simulink model "QN1F_induction_motor_v10"  (R2025b)
settings: Solver=ode45  StartTime=0.0  StopTime=10  RelTol=1e-3
PreLoadFcn:
  | run('QN1F_params_v10.m')
StopFcn:
  | QN1F_plot_results_v10
values from neighbouring files (symbols this model uses):
  B = 2.0e-5    (= 2e-05)    [QN1F_params_v10.m]
  f_max = n_max*pole_pairs/60    (= 400)    [QN1F_params_v10.m]
  I_rated = 10    [QN1F_params_v10.m]
  J = 2.5e-3    (= 0.0025)    [QN1F_params_v10.m]
  K_slip = T_rated/s_ref_model    (= 115)    [QN1F_params_v10.m]
  Kp_f = 0.05    [QN1F_params_v10.m]
  n_max = 24000    [QN1F_params_v10.m]
  n_ref = n_rated    (= 18000)    [QN1F_params_v10.m]
  pole_pairs = 1    [QN1F_params_v10.m]
  T_cut_amp = 0.15    [QN1F_params_v10.m]
  T_cut_mean = 1.0    (= 1)    [QN1F_params_v10.m]
  t_cut_start = 4.0    (= 4)    [QN1F_params_v10.m]
  T_rated = 2.3    [QN1F_params_v10.m]
  tau_T = 0.05    [QN1F_params_v10.m]
  w_tooth = 2*pi*f_tooth    (= 3769.91118431)    [QN1F_params_v10.m]
settings Model: Creator=jaxja  LastModifiedBy=jaxja
settings DataIOCC: ReturnWorkspaceOutputs=off

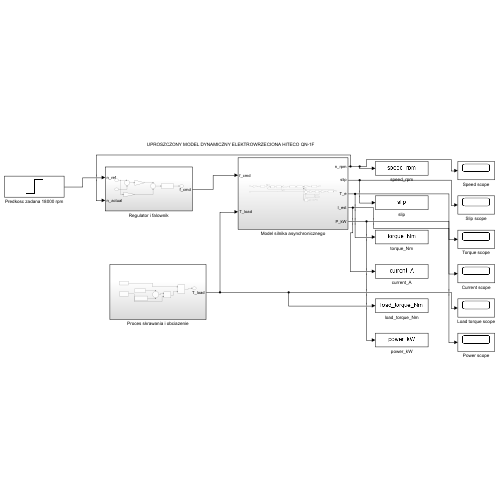
[thumbnail: Simulink's stored preview of the top-level diagram]
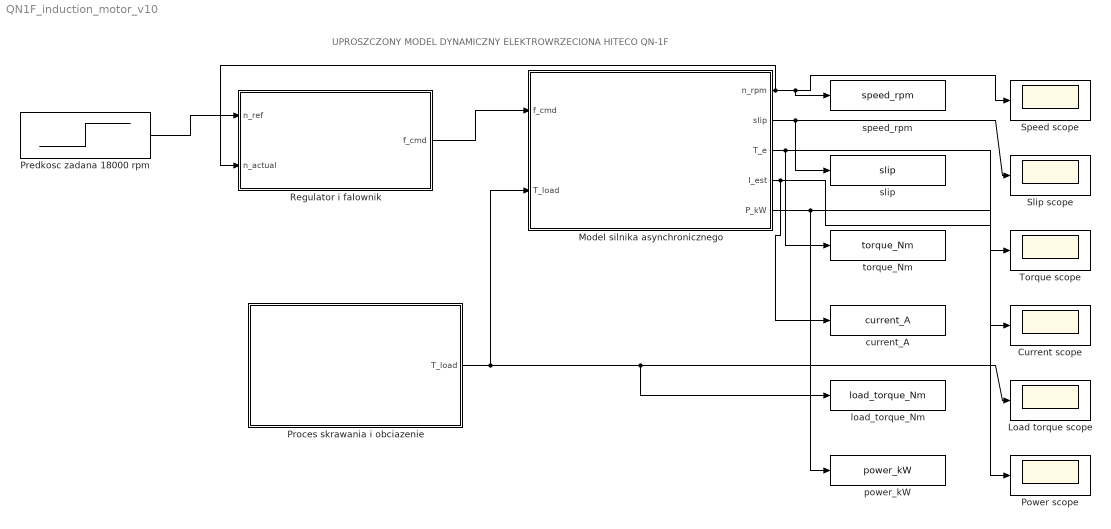
== system QN1F_induction_motor_v10 ==
  note: UPROSZCZONY MODEL DYNAMICZNY ELEKTROWRZECIONA HITECO QN-1F
  Current scope : Scope
  Load torque scope : Scope
  Model silnika asynchronicznego : Subsystem
  Power scope : Scope
  Predkosc zadana 18000 rpm : Step  Time=0.2  After=n_ref  SampleTime=0
  Proces skrawania i obciazenie : Subsystem
  Regulator i falownik : Subsystem
  Slip scope : Scope
  Speed scope : Scope
  Torque scope : Scope
  current_A : ToWorkspace  VariableName=current_A  SaveFormat=Timeseries  SampleTime=-1
  load_torque_Nm : ToWorkspace  VariableName=load_torque_Nm  SaveFormat=Timeseries  SampleTime=-1
  power_kW : ToWorkspace  VariableName=power_kW  SaveFormat=Timeseries  SampleTime=-1
  slip : ToWorkspace  VariableName=slip  SaveFormat=Timeseries  SampleTime=-1
  speed_rpm : ToWorkspace  VariableName=speed_rpm  SaveFormat=Timeseries  SampleTime=-1
  torque_Nm : ToWorkspace  VariableName=torque_Nm  SaveFormat=Timeseries  SampleTime=-1
  wires:
  Predkosc zadana 18000 rpm/1 -> Regulator i falownik/1(n_ref)
  Regulator i falownik/1(f_cmd) -> Model silnika asynchronicznego/1(f_cmd)
  Proces skrawania i obciazenie/1(T_load) -> load_torque_Nm/1, Load torque scope/1, Model silnika asynchronicznego/2(T_load)
  Model silnika asynchronicznego/1(n_rpm) -> speed_rpm/1, Speed scope/1, Regulator i falownik/2(n_actual)
  Model silnika asynchronicznego/2(slip) -> slip/1, Slip scope/1
  Model silnika asynchronicznego/3(T_e) -> torque_Nm/1, Torque scope/1
  Model silnika asynchronicznego/4(I_est) -> current_A/1, Current scope/1
  Model silnika asynchronicznego/5(P_kW) -> power_kW/1, Power scope/1

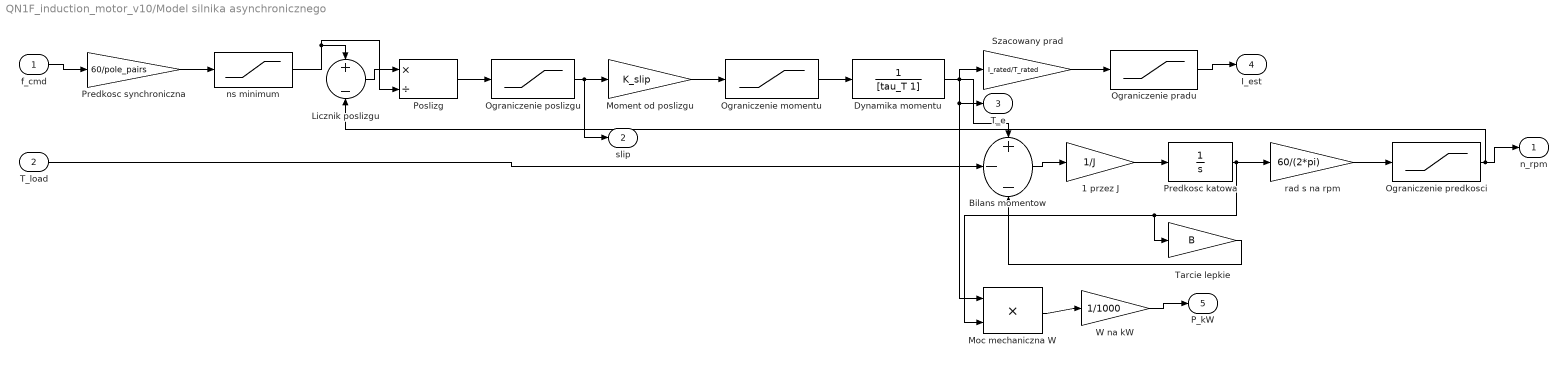
== system QN1F_induction_motor_v10/Model silnika asynchronicznego ==
  f_cmd : Inport
  T_load : Inport  Port=2
  1 przez J : Gain  Gain=1/J
  Bilans momentow : Sum  Inputs=+--
  Dynamika momentu : TransferFcn  Numerator=1  Denominator=[tau_T 1]
  Licznik poslizgu : Sum  Inputs=+-
  Moc mechaniczna W : Product
  Moment od poslizgu : Gain  Gain=K_slip
  Ograniczenie momentu : Saturate  UpperLimit=T_rated  LowerLimit=0
  Ograniczenie poslizgu : Saturate  UpperLimit=1  LowerLimit=0
  Ograniczenie pradu : Saturate  UpperLimit=I_rated  LowerLimit=0
  Ograniczenie predkosci : Saturate  UpperLimit=n_max  LowerLimit=0
  Poslizg : Product  Inputs=*/
  Predkosc katowa : Integrator
  Predkosc synchroniczna : Gain  Gain=60/pole_pairs
  Szacowany prad : Gain  Gain=I_rated/T_rated
  Tarcie lepkie : Gain  Gain=B
  W na kW : Gain  Gain=1/1000
  ns minimum : Saturate  UpperLimit=n_max  LowerLimit=1
  rad s na rpm : Gain  Gain=60/(2*pi)
  n_rpm : Outport
  slip : Outport  Port=2
  T_e : Outport  Port=3
  I_est : Outport  Port=4
  P_kW : Outport  Port=5
  wires:
  f_cmd/1 -> Predkosc synchroniczna/1
  Predkosc synchroniczna/1 -> ns minimum/1
  ns minimum/1 -> Licznik poslizgu/1, Poslizg/2
  Ograniczenie predkosci/1 -> Licznik poslizgu/2, n_rpm/1
  Licznik poslizgu/1 -> Poslizg/1
  Poslizg/1 -> Ograniczenie poslizgu/1
  Ograniczenie poslizgu/1 -> Moment od poslizgu/1, slip/1
  Moment od poslizgu/1 -> Ograniczenie momentu/1
  Ograniczenie momentu/1 -> Dynamika momentu/1
  Dynamika momentu/1 -> Moc mechaniczna W/1, T_e/1, Bilans momentow/1, Szacowany prad/1
  T_load/1 -> Bilans momentow/2
  Bilans momentow/1 -> 1 przez J/1
  1 przez J/1 -> Predkosc katowa/1
  Predkosc katowa/1 -> Tarcie lepkie/1, Moc mechaniczna W/2, rad s na rpm/1
  Tarcie lepkie/1 -> Bilans momentow/3
  rad s na rpm/1 -> Ograniczenie predkosci/1
  Szacowany prad/1 -> Ograniczenie pradu/1
  Moc mechaniczna W/1 -> W na kW/1
  Ograniczenie pradu/1 -> I_est/1
  W na kW/1 -> P_kW/1

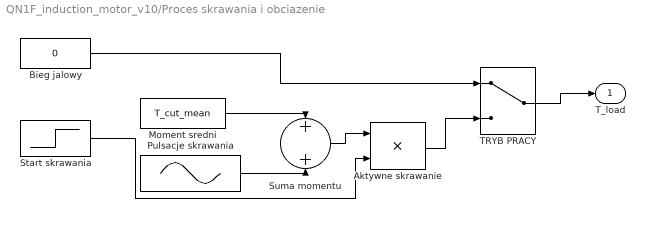
== system QN1F_induction_motor_v10/Proces skrawania i obciazenie ==
  Aktywne skrawanie : Product
  Bieg jalowy : Constant  Value=0
  Moment sredni : Constant  Value=T_cut_mean
  Pulsacje skrawania : Sin  Amplitude=T_cut_amp  Frequency=w_tooth  SampleTime=0
  Start skrawania : Step  Time=t_cut_start  SampleTime=0
  Suma momentu : Sum
  TRYB PRACY : ManualSwitch
  T_load : Outport
  wires:
  Moment sredni/1 -> Suma momentu/1
  Pulsacje skrawania/1 -> Suma momentu/2
  Suma momentu/1 -> Aktywne skrawanie/1
  Start skrawania/1 -> Aktywne skrawanie/2
  Bieg jalowy/1 -> TRYB PRACY/1
  Aktywne skrawanie/1 -> TRYB PRACY/2
  TRYB PRACY/1 -> T_load/1

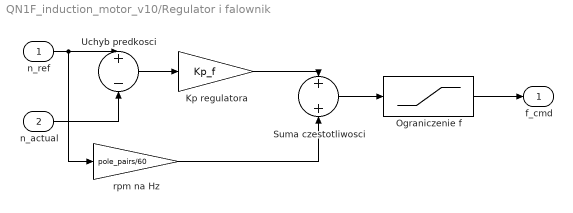
== system QN1F_induction_motor_v10/Regulator i falownik ==
  n_ref : Inport
  n_actual : Inport  Port=2
  Kp regulatora : Gain  Gain=Kp_f
  Ograniczenie f : Saturate  UpperLimit=f_max  LowerLimit=0
  Suma czestotliwosci : Sum
  Uchyb predkosci : Sum  Inputs=+-
  rpm na Hz : Gain  Gain=pole_pairs/60
  f_cmd : Outport
  wires:
  n_ref/1 -> Uchyb predkosci/1, rpm na Hz/1
  n_actual/1 -> Uchyb predkosci/2
  Uchyb predkosci/1 -> Kp regulatora/1
  Kp regulatora/1 -> Suma czestotliwosci/1
  rpm na Hz/1 -> Suma czestotliwosci/2
  Suma czestotliwosci/1 -> Ograniczenie f/1
  Ograniczenie f/1 -> f_cmd/1
